simulink model "AXI_QPSK_Tx"  (R2023b)
settings: Solver=FixedStepAuto  StartTime=0.0  StopTime=10/Rb  RelTol=1e-3
PreLoadFcn:
  | Rb = 1000;   % 1kbit / s
  | Rsym = Rb/2;   % 2 bits per symbol
  | Rsymbol = Rb/2;
  | OSR = 32;
  | f_error = 120;
  | 
  | design_filters_tx
values from neighbouring files (symbols this model uses):
  CIC_fine_Tx = 2^-(CIC_right_shift - CIC_left_shift - CIC_shift_Tx)    [design_filters_tx.m]
  fCIC = fCICcomp * R_CIC    (= 25600000)    [design_filters_tx.m]
  fHB = fRRC * R_HB    (= 4000)    [design_filters_tx.m]
  R_CIC = 3200    [design_filters_tx.m]
  R_CICcomp = 2    [design_filters_tx.m]
  R_HB = 2    [design_filters_tx.m]
  R_RRC = 4    [design_filters_tx.m]
undefined symbols (not defined in the file or in its folder): AXI4, Lite
libraries: hdlBasic x309, hdlDSPIP x8, hdlsllib x2, vmcUtilities x1
(part 1 of 3)
CloseFcn:
  | clear
settings Model: Creator=nas07122  LastModifiedBy=Jakub
settings SolverCC: AlgebraicLoopSolver=TrustRegion
settings DataIOCC: ReturnWorkspaceOutputs=off
settings DebuggingCC: UnconnectedInputMsg=warning  UnconnectedOutputMsg=warning  UnconnectedLineMsg=warning  ArithmeticOperatorsInVariantConditions=warning
settings ModelReferenceCC: EnableRefExpFcnMdlSchedulingChecks=on
settings SFSimCC: SimUseLocalCustomCode=off  CustomCodeUndefinedFunction=UseInterfaceOnly
settings RTWCC: RTWUseLocalCustomCode=off
settings CodeAppCC: StateflowObjectComments=on

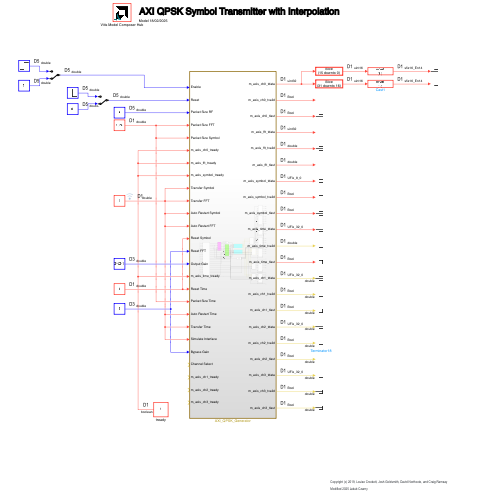
[thumbnail: Simulink's stored preview of the top-level diagram]
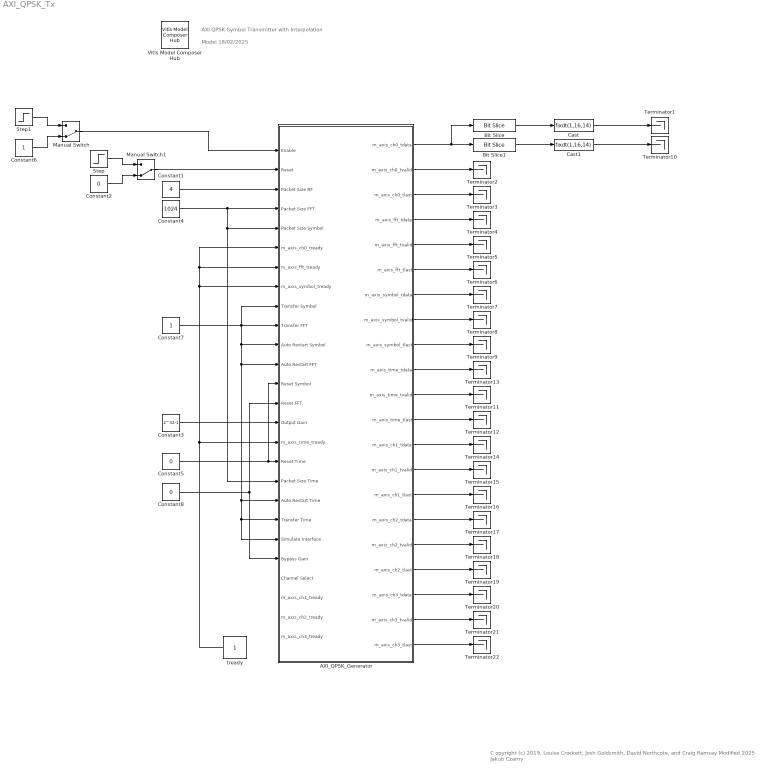
== system AXI_QPSK_Tx ==
  note: Model 18/02/2025
  note: AXI QPSK Symbol Transmitter with Interpolation
  note: C opyright (c) 2019, Louise Crockett, Josh Goldsmith, David Northcote, and Craig Ramsay
      | Modified 2025 Jakub Czarny
  AXI_QPSK_Generator : Subsystem
  Bit Slice : hdlsllib/Logic and Bit Operations/Bit Slice  lidx=15  ridx=0
  Bit Slice1 : hdlsllib/Logic and Bit Operations/Bit Slice  lidx=31  ridx=16
  Cast : DataTypeConversion  OutDataTypeStr=fixdt(1,16,14)  ConvertRealWorld=Stored Integer (SI)  SaturateOnIntegerOverflow=off  RndMeth=Floor
  Cast1 : DataTypeConversion  OutDataTypeStr=fixdt(1,16,14)  ConvertRealWorld=Stored Integer (SI)  SaturateOnIntegerOverflow=off  RndMeth=Floor
  Constant1 : Constant  Value=4  SampleTime=2/Rb
  Constant2 : Constant  Value=0  SampleTime=2/Rb
  Constant3 : Constant  Value=2^32-1  SampleTime=1/fHB
  Constant4 : Constant  Value=1024  SampleTime=1/fCIC
  Constant5 : Constant  Value=0  SampleTime=1/fCIC
  Constant6 : Constant  SampleTime=2/Rb
  Constant7 : Constant  SampleTime=1/fCIC
  Constant8 : Constant  Value=0  SampleTime=1/fHB
  Manual Switch : ManualSwitch  CurrentSetting=0
  Manual Switch1 : ManualSwitch  CurrentSetting=0
  Step : Step  Time=5/Rb  Before=1  After=0  SampleTime=2/Rb
  Step1 : Step  Time=8/Rb  SampleTime=2/Rb
  Terminator{1..22} (22 alike) : Terminator
  Vitis Model Composer Hub : vmcUtilities/Vitis Model Composer Hub  Tag=genX  CodeGeneration=off  SubsystemName=AXI_QPSK_Tx  CompilationType=HDLCompilation  ExportTypeV2=IP Catalog  TargetDirectory=../iprepo/zcu111/tx  exportDesign=off  analyzeDesign=off  validateDesignOnHw=off  ExportType=System Generator  IpVendor=xilinx.com  IpLibrary=hls  IpVersion=1.0  IpHWLanguage=Verilog  AieCompilerOptions={}  AieSimulatorOptions={}  CreateTestbench=off  TestbenchStackSize=10  RunRtlSim=off  RunCSim=off  RunAieSim=off  AieSimTimeout=50000  RunAieSimProfiling=off  LaunchVitisAnalyzer=off  PlotOutput=off  RunX86Sim=off  X86SimTimeout=10  GenHwImage=off  GenLibadfXo=on  GenHwValidationCode=off  PlatformType=Not Specified  HwSystemType=Baremetal  HwValidationTarget=hw  ProjDevice=xczu28dr-ffvg1517-2-e  ProjDevicePart=xczu28dr-ffvg1517-2-e  SamplePeriod=-1  ClockFrequency=200  DataPathParallelism=1  xilinxfamily=zynquplusRFSOC  part=xczu28dr  speed=-2-e  package=ffvg1517  directory=../iprepo/zcu111/tx\ip\AXI_QPSK_Tx\src  testbench=off  incr_netlist=off  synthesis_tool=Vivado  clock_wrapper=Clock Enables  dbl_ovrd=According to Block Masks  dcm_input_clock_period=10  sysclk_period=(1/fCIC)*1e9  simulink_period=1/(0.5*Rb*R_RRC*R_HB*R_CICcomp*R_CIC)  eval_field=0  LogFileName=''  NThreads=4
  tready : Constant  VectorParams1D=off  OutDataTypeStr=boolean  SampleTime=-1
  wires:
  Step1/1 -> Manual Switch/1
  Constant6/1 -> Manual Switch/2
  Bit Slice/1 -> Cast/1
  Bit Slice1/1 -> Cast1/1
  AXI_QPSK_Generator/1(m_axis_ch0_tdata) -> Bit Slice/1, Bit Slice1/1
  Manual Switch/1 -> AXI_QPSK_Generator/1(Enable)
  Constant1/1 -> AXI_QPSK_Generator/3(Packet Size RF)
  tready/1 -> AXI_QPSK_Generator/7(m_axis_fft_tready), AXI_QPSK_Generator/6(m_axis_ch0_tready), AXI_QPSK_Generator/8(m_axis_symbol_tready), AXI_QPSK_Generator/16(m_axis_time_tready)
  Manual Switch1/1 -> AXI_QPSK_Generator/2(Reset)
  Step/1 -> Manual Switch1/1
  Constant2/1 -> Manual Switch1/2
  Constant4/1 -> AXI_QPSK_Generator/5(Packet Size Symbol), AXI_QPSK_Generator/18(Packet Size Time), AXI_QPSK_Generator/4(Packet Size FFT)
  Constant5/1 -> AXI_QPSK_Generator/13(Reset Symbol), AXI_QPSK_Generator/17(Reset Time)
  Constant7/1 -> AXI_QPSK_Generator/21(Simulate Interface), AXI_QPSK_Generator/20(Transfer Time), AXI_QPSK_Generator/19(Auto Restart Time), AXI_QPSK_Generator/12(Auto Restart FFT), AXI_QPSK_Generator/11(Auto Restart Symbol), AXI_QPSK_Generator/10(Transfer FFT), AXI_QPSK_Generator/9(Transfer Symbol)
  Constant8/1 -> AXI_QPSK_Generator/14(Reset FFT), AXI_QPSK_Generator/22(Bypass Gain)
  Constant3/1 -> AXI_QPSK_Generator/15(Output Gain)
  AXI_QPSK_Generator/2(m_axis_ch0_tvalid) -> Terminator2/1
  AXI_QPSK_Generator/3(m_axis_ch0_tlast) -> Terminator3/1
  AXI_QPSK_Generator/5(m_axis_fft_tvalid) -> Terminator5/1
  AXI_QPSK_Generator/4(m_axis_fft_tdata) -> Terminator4/1
  AXI_QPSK_Generator/8(m_axis_symbol_tvalid) -> Terminator8/1
  AXI_QPSK_Generator/9(m_axis_symbol_tlast) -> Terminator9/1
  AXI_QPSK_Generator/7(m_axis_symbol_tdata) -> Terminator7/1
  AXI_QPSK_Generator/6(m_axis_fft_tlast) -> Terminator6/1
  AXI_QPSK_Generator/12(m_axis_time_tlast) -> Terminator12/1
  AXI_QPSK_Generator/10(m_axis_time_tdata) -> Terminator13/1
  Cast/1 -> Terminator1/1
  Cast1/1 -> Terminator10/1
  AXI_QPSK_Generator/11(m_axis_time_tvalid) -> Terminator11/1
  AXI_QPSK_Generator/13(m_axis_ch1_tdata) -> Terminator14/1
  AXI_QPSK_Generator/14(m_axis_ch1_tvalid) -> Terminator15/1
  AXI_QPSK_Generator/15(m_axis_ch1_tlast) -> Terminator16/1
  AXI_QPSK_Generator/16(m_axis_ch2_tdata) -> Terminator17/1
  AXI_QPSK_Generator/17(m_axis_ch2_tvalid) -> Terminator18/1
  AXI_QPSK_Generator/18(m_axis_ch2_tlast) -> Terminator19/1
  AXI_QPSK_Generator/19(m_axis_ch3_tdata) -> Terminator20/1
  AXI_QPSK_Generator/20(m_axis_ch3_tvalid) -> Terminator21/1
  AXI_QPSK_Generator/21(m_axis_ch3_tlast) -> Terminator22/1

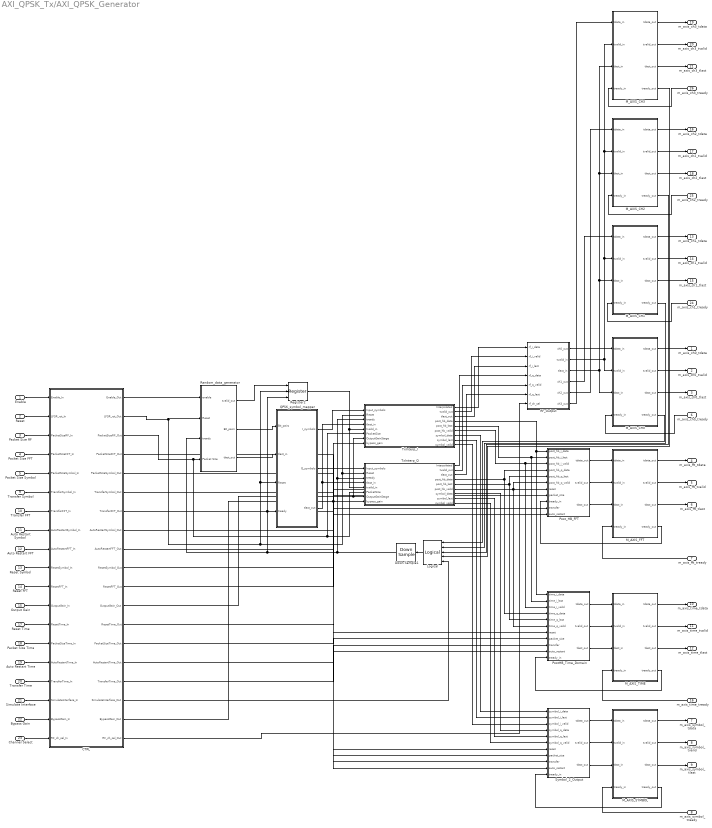
== system AXI_QPSK_Tx/AXI_QPSK_Generator ==
  Enable : Inport
  Reset : Inport  Port=2
  Packet Size RF : Inport  Port=3
  Packet Size FFT : Inport  Port=4
  Packet Size Symbol : Inport  Port=5
  m_axis_ch0_tready : Inport  Port=6
  m_axis_fft_tready : Inport  Port=7
  m_axis_symbol_tready : Inport  Port=8
  Transfer Symbol : Inport  Port=9
  Transfer FFT : Inport  Port=10
  Auto Restart Symbol : Inport  Port=11
  Auto Restart FFT : Inport  Port=12
  Reset Symbol : Inport  Port=13
  Reset FFT : Inport  Port=14
  Output Gain : Inport  Port=15
  m_axis_time_tready : Inport  Port=16
  Reset Time : Inport  Port=17
  Packet Size Time : Inport  Port=18
  Auto Restart Time : Inport  Port=19
  Transfer Time : Inport  Port=20
  Simulate Interface : Inport  Port=21
  Bypass Gain : Inport  Port=22
  Channel Select : Inport  Port=23
  m_axis_ch1_tready : Inport  Port=24
  m_axis_ch2_tready : Inport  Port=25
  m_axis_ch3_tready : Inport  Port=26
  CTRL : Subsystem
  Down Sample1 : hdlBasic/Down Sample  sample_ratio=fCIC/(Rb/2)  sample_phase=First Value of Frame  en=off  rst=off  latency=0  XmcBlockStatus=1  maskContainerNames=group1  block_type=dsamp  block_config=sysgen:Downsample_config
  Logical : hdlBasic/Logical  logical_function=OR  inputs=5  en=off  latency=0  precision=Full  arith_type=Unsigned  n_bits=16  bin_pt=0  align_bp=on  overflow=[]  quantization=[]  XmcBlockStatus=1  maskContainerNames=tabcontainer1  block_type=logical  block_config=sysgen:Logical_config
  M_AXIS_CH0 : Subsystem
  M_AXIS_CH1 : Subsystem
  M_AXIS_CH2 : Subsystem
  M_AXIS_CH3 : Subsystem
  M_AXIS_FFT : Subsystem
  M_AXIS_SYMBOL : Subsystem
  M_AXIS_TIME : Subsystem
  PostHB_Time_Domain : Subsystem
  Post_HB_FFT : Subsystem
  QPSK_symbol_mapper : Subsystem
  RF_Output : Subsystem
  Random_data_generator : Subsystem
  Register2 : hdlBasic/Register  init=0  rst=on  en=on  XmcBlockStatus=1  maskContainerNames=tabcontainer1  block_type=register  block_config=sysgen:Register_config
  Symbol_2_Output : Subsystem
  TxInterp_I : Subsystem
  TxInterp_Q : Subsystem
  m_axis_ch0_tdata : Outport  VectorParamsAs1DForOutWhenUnconnected=off
  m_axis_ch0_tvalid : Outport  Port=2  VectorParamsAs1DForOutWhenUnconnected=off
  m_axis_ch0_tlast : Outport  Port=3  VectorParamsAs1DForOutWhenUnconnected=off
  m_axis_fft_tdata : Outport  Port=4  VectorParamsAs1DForOutWhenUnconnected=off
  m_axis_fft_tvalid : Outport  Port=5  VectorParamsAs1DForOutWhenUnconnected=off
  m_axis_fft_tlast : Outport  Port=6  VectorParamsAs1DForOutWhenUnconnected=off
  m_axis_symbol_tdata : Outport  Port=7  VectorParamsAs1DForOutWhenUnconnected=off
  m_axis_symbol_tvalid : Outport  Port=8  VectorParamsAs1DForOutWhenUnconnected=off
  m_axis_symbol_tlast : Outport  Port=9  VectorParamsAs1DForOutWhenUnconnected=off
  m_axis_time_tdata : Outport  Port=10  VectorParamsAs1DForOutWhenUnconnected=off
  m_axis_time_tvalid : Outport  Port=11  VectorParamsAs1DForOutWhenUnconnected=off
  m_axis_time_tlast : Outport  Port=12  VectorParamsAs1DForOutWhenUnconnected=off
  m_axis_ch1_tdata : Outport  Port=13  VectorParamsAs1DForOutWhenUnconnected=off
  m_axis_ch1_tvalid : Outport  Port=14  VectorParamsAs1DForOutWhenUnconnected=off
  m_axis_ch1_tlast : Outport  Port=15  VectorParamsAs1DForOutWhenUnconnected=off
  m_axis_ch2_tdata : Outport  Port=16  VectorParamsAs1DForOutWhenUnconnected=off
  m_axis_ch2_tvalid : Outport  Port=17  VectorParamsAs1DForOutWhenUnconnected=off
  m_axis_ch2_tlast : Outport  Port=18  VectorParamsAs1DForOutWhenUnconnected=off
  m_axis_ch3_tdata : Outport  Port=19  VectorParamsAs1DForOutWhenUnconnected=off
  m_axis_ch3_tvalid : Outport  Port=20  VectorParamsAs1DForOutWhenUnconnected=off
  m_axis_ch3_tlast : Outport  Port=21  VectorParamsAs1DForOutWhenUnconnected=off
  wires:
  QPSK_symbol_mapper/3(tlast_out) -> TxInterp_I/4(tlast_in), TxInterp_Q/4(tlast_in)
  M_AXIS_CH0/2(tvalid_out) -> m_axis_ch0_tvalid/1
  QPSK_symbol_mapper/1(I_symbols) -> TxInterp_I/1(Input_symbols)
  m_axis_ch0_tready/1 -> M_AXIS_CH0/4(tready_in)
  QPSK_symbol_mapper/2(Q_symbols) -> TxInterp_Q/1(Input_symbols)
  Packet Size RF/1 -> CTRL/3(PacketSizeRF_In)
  Reset/1 -> CTRL/2(LFSR_rst_In)
  Random_data_generator/3(tlast_out) -> QPSK_symbol_mapper/2(tlast_in)
  Enable/1 -> CTRL/1(Enable_In)
  Random_data_generator/2(Bit_pairs) -> QPSK_symbol_mapper/1(Bit_pairs)
  CTRL/3(PacketSizeRF_Out) -> TxInterp_I/6(PacketSize), TxInterp_Q/6(PacketSize), Random_data_generator/4(Packet Size)
  M_AXIS_CH0/3(tlast_out) -> m_axis_ch0_tlast/1
  M_AXIS_CH0/1(tdata_out) -> m_axis_ch0_tdata/1
  Down Sample1/1 -> Random_data_generator/3(tready), Register2/3, QPSK_symbol_mapper/4(tready), TxInterp_I/3(tready), TxInterp_Q/3(tready)
  CTRL/2(LFSR_rst_Out) -> Random_data_generator/2(Reset), TxInterp_I/2(Reset), TxInterp_Q/2(Reset), QPSK_symbol_mapper/3(Reset), Register2/2
  CTRL/1(Enable_Out) -> Random_data_generator/1(enable)
  Random_data_generator/1(tvalid_out) -> Register2/1
  Register2/1 -> TxInterp_I/5(tvalid_in), TxInterp_Q/5(tvalid_in)
  Post_HB_FFT/1(tdata_out) -> M_AXIS_FFT/1(tdata_in)
  Post_HB_FFT/2(tvalid_out) -> M_AXIS_FFT/2(tvalid_in)
  Post_HB_FFT/3(tlast_out) -> M_AXIS_FFT/3(tlast_in)
  M_AXIS_FFT/1(tdata_out) -> m_axis_fft_tdata/1
  M_AXIS_FFT/3(tlast_out) -> m_axis_fft_tlast/1
  m_axis_fft_tready/1 -> M_AXIS_FFT/4(tready_in)
  M_AXIS_FFT/2(tvalid_out) -> m_axis_fft_tvalid/1
  M_AXIS_SYMBOL/2(tvalid_out) -> m_axis_symbol_tvalid/1
  m_axis_symbol_tready/1 -> M_AXIS_SYMBOL/4(tready_in)
  M_AXIS_SYMBOL/3(tlast_out) -> m_axis_symbol_tlast/1
  M_AXIS_SYMBOL/1(tdata_out) -> m_axis_symbol_tdata/1
  TxInterp_I/4(post_hb_data) -> PostHB_Time_Domain/1(time_i_data), Post_HB_FFT/1(post_hb_i_data)
  TxInterp_I/5(post_hb_last) -> PostHB_Time_Domain/2(time_i_last), Post_HB_FFT/2(post_hb_i_last)
  TxInterp_I/6(post_hb_valid) -> PostHB_Time_Domain/3(time_i_valid), Post_HB_FFT/3(post_hb_i_valid)
  Symbol_2_Output/1(tdata_out) -> M_AXIS_SYMBOL/1(tdata_in)
  Symbol_2_Output/2(tvalid_out) -> M_AXIS_SYMBOL/2(tvalid_in)
  Symbol_2_Output/3(tlast_out) -> M_AXIS_SYMBOL/3(tlast_in)
  M_AXIS_SYMBOL/4(tready_out) -> Symbol_2_Output/11(tready_in)
  M_AXIS_FFT/4(tready_out) -> Post_HB_FFT/9(tready_in)
  TxInterp_I/1(Interpolated) -> RF_Output/1(rf_i_data)
  TxInterp_I/2(tvalid_out) -> RF_Output/2(rf_i_valid)
  TxInterp_I/3(tlast_out) -> RF_Output/3(rf_i_last)
  RF_Output/1(ch0_out) -> M_AXIS_CH0/1(tdata_in)
  RF_Output/2(tvalid_in) -> M_AXIS_CH0/2(tvalid_in), M_AXIS_CH3/2(tvalid_in), M_AXIS_CH2/2(tvalid_in), M_AXIS_CH1/2(tvalid_in)
  RF_Output/3(tlast_in) -> M_AXIS_CH3/3(tlast_in), M_AXIS_CH2/3(tlast_in), M_AXIS_CH1/3(tlast_in), M_AXIS_CH0/3(tlast_in)
  TxInterp_I/7(symbol_data) -> Symbol_2_Output/1(symbol_i_data)
  TxInterp_I/8(symbol_last) -> Symbol_2_Output/2(symbol_i_last)
  TxInterp_I/9(symbol_valid) -> Symbol_2_Output/3(symbol_i_valid)
  CTRL/4(PacketSizeFFT_Out) -> Post_HB_FFT/8(packet_size)
  CTRL/5(PacketSizeSymbol_Out) -> Symbol_2_Output/8(packet_size)
  Packet Size FFT/1 -> CTRL/4(PacketSizeFFT_In)
  Packet Size Symbol/1 -> CTRL/5(PacketSizeSymbol_In)
  CTRL/6(TransferSymbol_Out) -> Symbol_2_Output/9(transfer)
  CTRL/8(AutoRestartSymbol_Out) -> Symbol_2_Output/10(auto_restart)
  CTRL/10(ResetSymbol_Out) -> Symbol_2_Output/7(reset)
  Transfer Symbol/1 -> CTRL/6(TransferSymbol_In)
  Transfer FFT/1 -> CTRL/7(TransferFFT_In)
  Auto Restart Symbol/1 -> CTRL/8(AutoRestartSymbol_In)
  Auto Restart FFT/1 -> CTRL/9(AutoRestartFFT_In)
  Reset Symbol/1 -> CTRL/10(ResetSymbol_In)
  Reset FFT/1 -> CTRL/11(ResetFFT_In)
  CTRL/7(TransferFFT_Out) -> Post_HB_FFT/10(transfer)
  CTRL/9(AutoRestartFFT_Out) -> Post_HB_FFT/11(auto_restart)
  CTRL/11(ResetFFT_Out) -> Post_HB_FFT/7(reset)
  CTRL/12(OutputGain_Out) -> TxInterp_I/7(OutputGainStage), TxInterp_Q/7(OutputGainStage)
  Output Gain/1 -> CTRL/12(OutputGain_In)
  M_AXIS_TIME/4(tready_out) -> PostHB_Time_Domain/11(tready_in)
  PostHB_Time_Domain/3(tlast_out) -> M_AXIS_TIME/3(tlast_in)
  PostHB_Time_Domain/2(tvalid_out) -> M_AXIS_TIME/2(tvalid_in)
  PostHB_Time_Domain/1(tdata_out) -> M_AXIS_TIME/1(tdata_in)
  M_AXIS_TIME/1(tdata_out) -> m_axis_time_tdata/1
  M_AXIS_TIME/3(tlast_out) -> m_axis_time_tlast/1
  m_axis_time_tready/1 -> M_AXIS_TIME/4(tready_in)
  M_AXIS_TIME/2(tvalid_out) -> m_axis_time_tvalid/1
  CTRL/13(ResetTime_Out) -> PostHB_Time_Domain/7(reset)
  CTRL/14(PacketSizeTime_Out) -> PostHB_Time_Domain/8(packet_size)
  CTRL/15(AutoRestartTime_Out) -> PostHB_Time_Domain/10(auto_restart)
  CTRL/16(TransferTime_Out) -> PostHB_Time_Domain/9(transfer)
  Reset Time/1 -> CTRL/13(ResetTime_In)
  Packet Size Time/1 -> CTRL/14(PacketSizeTime_In)
  Auto Restart Time/1 -> CTRL/15(AutoRestartTime_In)
  Transfer Time/1 -> CTRL/16(TransferTime_In)
  M_AXIS_CH0/4(tready_out) -> Logical/1
  Logical/1 -> Down Sample1/1
  CTRL/17(SimulateInterface_Out) -> Logical/5
  Simulate Interface/1 -> CTRL/17(SimulateInterface_In)
  CTRL/18(BypassGain_Out) -> TxInterp_I/8(bypass_gain), TxInterp_Q/8(bypass_gain)
  TxInterp_Q/1(Interpolated) -> RF_Output/4(rf_q_data)
  TxInterp_Q/2(tvalid_out) -> RF_Output/5(rf_q_valid)
  TxInterp_Q/3(tlast_out) -> RF_Output/6(rf_q_last)
  TxInterp_Q/4(post_hb_data) -> PostHB_Time_Domain/4(time_q_data), Post_HB_FFT/4(post_hb_q_data)
  TxInterp_Q/5(post_hb_last) -> PostHB_Time_Domain/5(time_q_last), Post_HB_FFT/5(post_hb_q_last)
  TxInterp_Q/6(post_hb_valid) -> PostHB_Time_Domain/6(time_q_valid), Post_HB_FFT/6(post_hb_q_valid)
  TxInterp_Q/7(symbol_data) -> Symbol_2_Output/4(symbol_q_data)
  TxInterp_Q/8(symbol_last) -> Symbol_2_Output/5(symbol_q_last)
  TxInterp_Q/9(symbol_valid) -> Symbol_2_Output/6(symbol_q_valid)
  Bypass Gain/1 -> CTRL/18(BypassGain_In)
  Channel Select/1 -> CTRL/19(RF_ch_sel_In)
  CTRL/19(RF_ch_sel_Out) -> RF_Output/7(rf_ch_sel)
  M_AXIS_CH1/3(tlast_out) -> m_axis_ch1_tlast/1
  M_AXIS_CH1/1(tdata_out) -> m_axis_ch1_tdata/1
  m_axis_ch1_tready/1 -> M_AXIS_CH1/4(tready_in)
  M_AXIS_CH1/2(tvalid_out) -> m_axis_ch1_tvalid/1
  M_AXIS_CH1/4(tready_out) -> Logical/2
  RF_Output/4(ch1_out) -> M_AXIS_CH1/1(tdata_in)
  M_AXIS_CH2/2(tvalid_out) -> m_axis_ch2_tvalid/1
  M_AXIS_CH2/1(tdata_out) -> m_axis_ch2_tdata/1
  m_axis_ch2_tready/1 -> M_AXIS_CH2/4(tready_in)
  M_AXIS_CH2/3(tlast_out) -> m_axis_ch2_tlast/1
  RF_Output/5(ch2_out) -> M_AXIS_CH2/1(tdata_in)
  M_AXIS_CH2/4(tready_out) -> Logical/3
  m_axis_ch3_tready/1 -> M_AXIS_CH3/4(tready_in)
  M_AXIS_CH3/1(tdata_out) -> m_axis_ch3_tdata/1
  M_AXIS_CH3/2(tvalid_out) -> m_axis_ch3_tvalid/1
  M_AXIS_CH3/3(tlast_out) -> m_axis_ch3_tlast/1
  M_AXIS_CH3/4(tready_out) -> Logical/4
  RF_Output/6(ch3_out) -> M_AXIS_CH3/1(tdata_in)

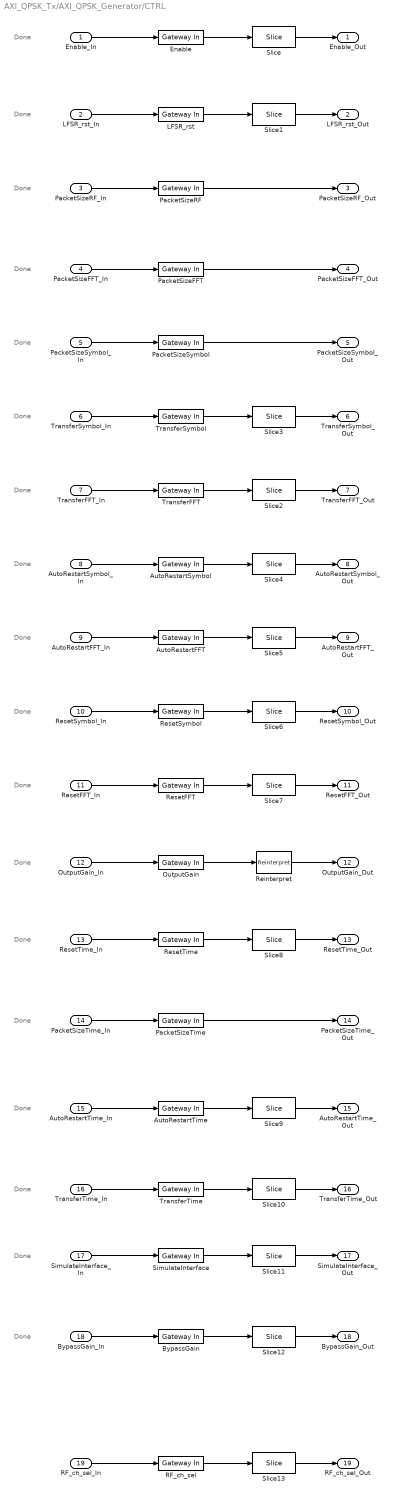
== system AXI_QPSK_Tx/AXI_QPSK_Generator/CTRL ==
  note: Done
  note: Done
  note: Done
  note: Done
  note: Done
  note: Done
  note: Done
  note: Done
  note: Done
  note: Done
  note: Done
  note: Done
  note: Done
  note: Done
  note: Done
  note: Done
  note: Done
  note: Done
  Enable_In : Inport
  LFSR_rst_In : Inport  Port=2
  PacketSizeRF_In : Inport  Port=3
  PacketSizeFFT_In : Inport  Port=4
  PacketSizeSymbol_In : Inport  Port=5
  TransferSymbol_In : Inport  Port=6
  TransferFFT_In : Inport  Port=7
  AutoRestartSymbol_In : Inport  Port=8
  AutoRestartFFT_In : Inport  Port=9
  ResetSymbol_In : Inport  Port=10
  ResetFFT_In : Inport  Port=11
  OutputGain_In : Inport  Port=12
  ResetTime_In : Inport  Port=13
  PacketSizeTime_In : Inport  Port=14
  AutoRestartTime_In : Inport  Port=15
  TransferTime_In : Inport  Port=16
  SimulateInterface_In : Inport  Port=17
  BypassGain_In : Inport  Port=18
  RF_ch_sel_In : Inport  Port=19
  AutoRestartFFT : hdlBasic/Gateway In  gui_display_data_type=Fixed-point  arith_type=Unsigned  n_bits=32  bin_pt=0  preci_type=Single  exp_width=8  frac_width=24  rows=1  columns=1  quantization=Truncate  overflow=Wrap  period=1/fCIC  UseAsADC=off  ADCChannel='1'  interface=AXI4-Lite  automatic_assignment=off  address_offset=40  intf_name=''  intf_description=''  default_value=0  timing_constraint=None  locs_specified=off  LOCs={}  io_standard={}  inherit_from_input=off  hdl_port=on  XmcBlockStatus=1  maskContainerNames=group4  block_type=gatewayin  block_config=sysgen:gateway_in_config  block_width_w=590  block_height_w=620  block_width=640  block_height=850
  AutoRestartSymbol : hdlBasic/Gateway In  gui_display_data_type=Fixed-point  arith_type=Unsigned  n_bits=32  bin_pt=0  preci_type=Single  exp_width=8  frac_width=24  rows=1  columns=1  quantization=Truncate  overflow=Wrap  period=1/fCIC  UseAsADC=off  ADCChannel='1'  interface=AXI4-Lite  automatic_assignment=off  address_offset=36  intf_name=''  intf_description=''  default_value=0  timing_constraint=None  locs_specified=off  LOCs={}  io_standard={}  inherit_from_input=off  hdl_port=on  XmcBlockStatus=1  maskContainerNames=group4  block_type=gatewayin  block_config=sysgen:gateway_in_config  block_width_w=590  block_height_w=620  block_width=640  block_height=850
  AutoRestartTime : hdlBasic/Gateway In  gui_display_data_type=Fixed-point  arith_type=Unsigned  n_bits=32  bin_pt=0  preci_type=Single  exp_width=8  frac_width=24  rows=1  columns=1  quantization=Truncate  overflow=Wrap  period=1/fCIC  UseAsADC=off  ADCChannel='1'  interface=AXI4-Lite  automatic_assignment=off  address_offset=56  intf_name=''  intf_description=''  default_value=0  timing_constraint=None  locs_specified=off  LOCs={}  io_standard={}  inherit_from_input=off  hdl_port=on  XmcBlockStatus=1  maskContainerNames=group4  block_type=gatewayin  block_config=sysgen:gateway_in_config  block_width_w=590  block_height_w=620  block_width=640  block_height=850
  BypassGain : hdlBasic/Gateway In  gui_display_data_type=Fixed-point  arith_type=Unsigned  n_bits=32  bin_pt=0  preci_type=Single  exp_width=8  frac_width=24  rows=1  columns=1  quantization=Truncate  overflow=Wrap  period=1/fHB  UseAsADC=off  ADCChannel='1'  interface=AXI4-Lite  automatic_assignment=off  address_offset=68  intf_name=''  intf_description=''  default_value=0  timing_constraint=None  locs_specified=off  LOCs={}  io_standard={}  inherit_from_input=off  hdl_port=on  XmcBlockStatus=1  maskContainerNames=group4  block_type=gatewayin  block_config=sysgen:gateway_in_config  block_width_w=590  block_height_w=620  block_width=640  block_height=850
  Enable : hdlBasic/Gateway In  gui_display_data_type=Fixed-point  arith_type=Unsigned  n_bits=32  bin_pt=0  preci_type=Single  exp_width=8  frac_width=24  rows=1  columns=1  quantization="Round  (unbiased: +/- Inf)"  overflow=Saturate  period=2/Rb  UseAsADC=off  ADCChannel='1'  interface=AXI4-Lite  automatic_assignment=off  address_offset=32  intf_name=''  intf_description=''  default_value=0  timing_constraint=None  locs_specified=off  LOCs={}  io_standard={}  inherit_from_input=off  hdl_port=on  XmcBlockStatus=1  maskContainerNames=group4  block_type=gatewayin  block_config=sysgen:gateway_in_config  block_width_w=590  block_height_w=620  block_width=640  block_height=850
  LFSR_rst : hdlBasic/Gateway In  gui_display_data_type=Fixed-point  arith_type=Unsigned  n_bits=32  bin_pt=0  preci_type=Single  exp_width=8  frac_width=24  rows=1  columns=1  quantization="Round  (unbiased: +/- Inf)"  overflow=Saturate  period=2/Rb  UseAsADC=off  ADCChannel='1'  interface=AXI4-Lite  automatic_assignment=off  address_offset=28  intf_name=''  intf_description=''  default_value=0  timing_constraint=None  locs_specified=off  LOCs={}  io_standard={}  inherit_from_input=off  hdl_port=on  XmcBlockStatus=1  maskContainerNames=group4  block_type=gatewayin  block_config=sysgen:gateway_in_config  block_width_w=590  block_height_w=620  block_width=640  block_height=850
  OutputGain : hdlBasic/Gateway In  gui_display_data_type=Fixed-point  arith_type=Unsigned  n_bits=32  bin_pt=0  preci_type=Single  exp_width=8  frac_width=24  rows=1  columns=1  quantization=Truncate  overflow=Wrap  period=1/fHB  UseAsADC=off  ADCChannel='1'  interface=AXI4-Lite  automatic_assignment=off  address_offset=44  intf_name=''  intf_description=''  default_value=0  timing_constraint=None  locs_specified=off  LOCs={}  io_standard={}  inherit_from_input=off  hdl_port=on  XmcBlockStatus=1  maskContainerNames=group4  block_type=gatewayin  block_config=sysgen:gateway_in_config  block_width_w=590  block_height_w=620  block_width=640  block_height=850
  PacketSizeFFT : hdlBasic/Gateway In  gui_display_data_type=Fixed-point  arith_type=Unsigned  n_bits=32  bin_pt=0  preci_type=Single  exp_width=8  frac_width=24  rows=1  columns=1  quantization=Truncate  overflow=Wrap  period=1/fCIC  UseAsADC=off  ADCChannel='1'  interface=AXI4-Lite  automatic_assignment=off  address_offset=24  intf_name=''  intf_description=''  default_value=0  timing_constraint=None  locs_specified=off  LOCs={}  io_standard={}  inherit_from_input=off  hdl_port=on  XmcBlockStatus=1  maskContainerNames=group4  block_type=gatewayin  block_config=sysgen:gateway_in_config  block_width_w=590  block_height_w=620  block_width=640  block_height=850
  PacketSizeRF : hdlBasic/Gateway In  gui_display_data_type=Fixed-point  arith_type=Unsigned  n_bits=32  bin_pt=0  preci_type=Single  exp_width=8  frac_width=24  rows=1  columns=1  quantization=Truncate  overflow=Wrap  period=2/Rb  UseAsADC=off  ADCChannel='1'  interface=AXI4-Lite  automatic_assignment=off  address_offset=20  intf_name=''  intf_description=''  default_value=0  timing_constraint=None  locs_specified=off  LOCs={}  io_standard={}  inherit_from_input=off  hdl_port=on  XmcBlockStatus=1  maskContainerNames=group4  block_type=gatewayin  block_config=sysgen:gateway_in_config  block_width_w=590  block_height_w=620  block_width=640  block_height=850
  PacketSizeSymbol : hdlBasic/Gateway In  gui_display_data_type=Fixed-point  arith_type=Unsigned  n_bits=32  bin_pt=0  preci_type=Single  exp_width=8  frac_width=24  rows=1  columns=1  quantization=Truncate  overflow=Wrap  period=1/fCIC  UseAsADC=off  ADCChannel='1'  interface=AXI4-Lite  automatic_assignment=off  address_offset=16  intf_name=''  intf_description=''  default_value=0  timing_constraint=None  locs_specified=off  LOCs={}  io_standard={}  inherit_from_input=off  hdl_port=on  XmcBlockStatus=1  maskContainerNames=group4  block_type=gatewayin  block_config=sysgen:gateway_in_config  block_width_w=590  block_height_w=620  block_width=640  block_height=850
  PacketSizeTime : hdlBasic/Gateway In  gui_display_data_type=Fixed-point  arith_type=Unsigned  n_bits=32  bin_pt=0  preci_type=Single  exp_width=8  frac_width=24  rows=1  columns=1  quantization=Truncate  overflow=Wrap  period=1/fCIC  UseAsADC=off  ADCChannel='1'  interface=AXI4-Lite  automatic_assignment=off  address_offset=52  intf_name=''  intf_description=''  default_value=0  timing_constraint=None  locs_specified=off  LOCs={}  io_standard={}  inherit_from_input=off  hdl_port=on  XmcBlockStatus=1  maskContainerNames=group4  block_type=gatewayin  block_config=sysgen:gateway_in_config  block_width_w=590  block_height_w=620  block_width=640  block_height=850
  RF_ch_sel : hdlBasic/Gateway In  gui_display_data_type=Fixed-point  arith_type=Unsigned  n_bits=32  bin_pt=0  preci_type=Single  exp_width=8  frac_width=24  rows=1  columns=1  quantization="Round  (unbiased: +/- Inf)"  overflow=Saturate  period=2/Rb  UseAsADC=off  ADCChannel='1'  interface=AXI4-Lite  automatic_assignment=off  address_offset=72  intf_name=''  intf_description=''  default_value=0  timing_constraint=None  locs_specified=off  LOCs={}  io_standard={}  inherit_from_input=off  hdl_port=on  XmcBlockStatus=1  maskContainerNames=group4  block_type=gatewayin  block_config=sysgen:gateway_in_config  block_width_w=590  block_height_w=620  block_width=640  block_height=850
  Reinterpret : hdlBasic/Reinterpret  force_arith_type=off  arith_type=Unsigned  force_bin_pt=on  bin_pt=32  XmcBlockStatus=1  maskContainerNames=group1  block_type=reinterpret  block_config=sysgen:Reinterpret_config
  ResetFFT : hdlBasic/Gateway In  gui_display_data_type=Fixed-point  arith_type=Unsigned  n_bits=32  bin_pt=0  preci_type=Single  exp_width=8  frac_width=24  rows=1  columns=1  quantization=Truncate  overflow=Wrap  period=1/fHB  UseAsADC=off  ADCChannel='1'  interface=AXI4-Lite  automatic_assignment=off  address_offset=12  intf_name=''  intf_description=''  default_value=0  timing_constraint=None  locs_specified=off  LOCs={}  io_standard={}  inherit_from_input=off  hdl_port=on  XmcBlockStatus=1  maskContainerNames=group4  block_type=gatewayin  block_config=sysgen:gateway_in_config  block_width_w=590  block_height_w=620  block_width=640  block_height=850
  ResetSymbol : hdlBasic/Gateway In  gui_display_data_type=Fixed-point  arith_type=Unsigned  n_bits=32  bin_pt=0  preci_type=Single  exp_width=8  frac_width=24  rows=1  columns=1  quantization=Truncate  overflow=Wrap  period=1/fCIC  UseAsADC=off  ADCChannel='1'  interface=AXI4-Lite  automatic_assignment=off  address_offset=8  intf_name=''  intf_description=''  default_value=0  timing_constraint=None  locs_specified=off  LOCs={}  io_standard={}  inherit_from_input=off  hdl_port=on  XmcBlockStatus=1  maskContainerNames=group4  block_type=gatewayin  block_config=sysgen:gateway_in_config  block_width_w=590  block_height_w=620  block_width=640  block_height=850
  ResetTime : hdlBasic/Gateway In  gui_display_data_type=Fixed-point  arith_type=Unsigned  n_bits=32  bin_pt=0  preci_type=Single  exp_width=8  frac_width=24  rows=1  columns=1  quantization=Truncate  overflow=Wrap  period=1/fCIC  UseAsADC=off  ADCChannel='1'  interface=AXI4-Lite  automatic_assignment=off  address_offset=48  intf_name=''  intf_description=''  default_value=0  timing_constraint=None  locs_specified=off  LOCs={}  io_standard={}  inherit_from_input=off  hdl_port=on  XmcBlockStatus=1  maskContainerNames=group4  block_type=gatewayin  block_config=sysgen:gateway_in_config  block_width_w=590  block_height_w=620  block_width=640  block_height=850
  SimulateInterface : hdlBasic/Gateway In  gui_display_data_type=Fixed-point  arith_type=Unsigned  n_bits=32  bin_pt=0  preci_type=Single  exp_width=8  frac_width=24  rows=1  columns=1  quantization=Truncate  overflow=Wrap  period=1/fCIC  UseAsADC=off  ADCChannel='1'  interface=AXI4-Lite  automatic_assignment=off  address_offset=64  intf_name=''  intf_description=''  default_value=0  timing_constraint=None  locs_specified=off  LOCs={}  io_standard={}  inherit_from_input=off  hdl_port=on  XmcBlockStatus=1  maskContainerNames=group4  block_type=gatewayin  block_config=sysgen:gateway_in_config  block_width_w=590  block_height_w=620  block_width=640  block_height=850
  Slice{,1..12} (13 alike) : hdlBasic/Slice  nbits=1  boolean_output=on  mode=Two Bit Locations  bit1=0  base1=LSB of Input  bit0=0  base0=LSB of Input  XmcBlockStatus=1  maskContainerNames=group1  block_type=slice  block_config=sysgen:Slice_config
  Slice13 : hdlBasic/Slice  nbits=2  boolean_output=off  mode=Lower Bit Location + Width  bit1=0  base1=LSB of Input  bit0=0  base0=LSB of Input  XmcBlockStatus=1  maskContainerNames=group1  block_type=slice  block_config=sysgen:Slice_config
  TransferFFT : hdlBasic/Gateway In  gui_display_data_type=Fixed-point  arith_type=Unsigned  n_bits=32  bin_pt=0  preci_type=Single  exp_width=8  frac_width=24  rows=1  columns=1  quantization=Truncate  overflow=Wrap  period=1/fCIC  UseAsADC=off  ADCChannel='1'  interface=AXI4-Lite  automatic_assignment=off  address_offset=4  intf_name=''  intf_description=''  default_value=0  timing_constraint=None  locs_specified=off  LOCs={}  io_standard={}  inherit_from_input=off  hdl_port=on  XmcBlockStatus=1  maskContainerNames=group4  block_type=gatewayin  block_config=sysgen:gateway_in_config  block_width_w=590  block_height_w=620  block_width=640  block_height=850
  TransferSymbol : hdlBasic/Gateway In  gui_display_data_type=Fixed-point  arith_type=Unsigned  n_bits=32  bin_pt=0  preci_type=Single  exp_width=8  frac_width=24  rows=1  columns=1  quantization=Truncate  overflow=Wrap  period=1/fCIC  UseAsADC=off  ADCChannel='1'  interface=AXI4-Lite  automatic_assignment=off  address_offset=0  intf_name=''  intf_description=''  default_value=0  timing_constraint=None  locs_specified=off  LOCs={}  io_standard={}  inherit_from_input=off  hdl_port=on  XmcBlockStatus=1  maskContainerNames=group4  block_type=gatewayin  block_config=sysgen:gateway_in_config  block_width_w=590  block_height_w=620  block_width=640  block_height=850
  TransferTime : hdlBasic/Gateway In  gui_display_data_type=Fixed-point  arith_type=Unsigned  n_bits=32  bin_pt=0  preci_type=Single  exp_width=8  frac_width=24  rows=1  columns=1  quantization=Truncate  overflow=Wrap  period=1/fCIC  UseAsADC=off  ADCChannel='1'  interface=AXI4-Lite  automatic_assignment=off  address_offset=60  intf_name=''  intf_description=''  default_value=0  timing_constraint=None  locs_specified=off  LOCs={}  io_standard={}  inherit_from_input=off  hdl_port=on  XmcBlockStatus=1  maskContainerNames=group4  block_type=gatewayin  block_config=sysgen:gateway_in_config  block_width_w=590  block_height_w=620  block_width=640  block_height=850
  Enable_Out : Outport  VectorParamsAs1DForOutWhenUnconnected=off
  LFSR_rst_Out : Outport  Port=2  VectorParamsAs1DForOutWhenUnconnected=off
  PacketSizeRF_Out : Outport  Port=3  VectorParamsAs1DForOutWhenUnconnected=off
  PacketSizeFFT_Out : Outport  Port=4  VectorParamsAs1DForOutWhenUnconnected=off
  PacketSizeSymbol_Out : Outport  Port=5  VectorParamsAs1DForOutWhenUnconnected=off
  TransferSymbol_Out : Outport  Port=6  VectorParamsAs1DForOutWhenUnconnected=off
  TransferFFT_Out : Outport  Port=7  VectorParamsAs1DForOutWhenUnconnected=off
  AutoRestartSymbol_Out : Outport  Port=8  VectorParamsAs1DForOutWhenUnconnected=off
  AutoRestartFFT_Out : Outport  Port=9  VectorParamsAs1DForOutWhenUnconnected=off
  ResetSymbol_Out : Outport  Port=10  VectorParamsAs1DForOutWhenUnconnected=off
  ResetFFT_Out : Outport  Port=11  VectorParamsAs1DForOutWhenUnconnected=off
  OutputGain_Out : Outport  Port=12  VectorParamsAs1DForOutWhenUnconnected=off
  ResetTime_Out : Outport  Port=13  VectorParamsAs1DForOutWhenUnconnected=off
  PacketSizeTime_Out : Outport  Port=14  VectorParamsAs1DForOutWhenUnconnected=off
  AutoRestartTime_Out : Outport  Port=15  VectorParamsAs1DForOutWhenUnconnected=off
  TransferTime_Out : Outport  Port=16  VectorParamsAs1DForOutWhenUnconnected=off
  SimulateInterface_Out : Outport  Port=17  VectorParamsAs1DForOutWhenUnconnected=off
  BypassGain_Out : Outport  Port=18  VectorParamsAs1DForOutWhenUnconnected=off
  RF_ch_sel_Out : Outport  Port=19  VectorParamsAs1DForOutWhenUnconnected=off
  wires:
  Enable/1 -> Slice/1
  LFSR_rst_In/1 -> LFSR_rst/1
  LFSR_rst/1 -> Slice1/1
  PacketSizeRF_In/1 -> PacketSizeRF/1
  Enable_In/1 -> Enable/1
  Slice/1 -> Enable_Out/1
  Slice1/1 -> LFSR_rst_Out/1
  PacketSizeRF/1 -> PacketSizeRF_Out/1
  PacketSizeFFT/1 -> PacketSizeFFT_Out/1
  PacketSizeFFT_In/1 -> PacketSizeFFT/1
  PacketSizeSymbol_In/1 -> PacketSizeSymbol/1
  PacketSizeSymbol/1 -> PacketSizeSymbol_Out/1
  TransferFFT/1 -> Slice2/1
  TransferFFT_In/1 -> TransferFFT/1
  TransferSymbol_In/1 -> TransferSymbol/1
  TransferSymbol/1 -> Slice3/1
  AutoRestartSymbol/1 -> Slice4/1
  AutoRestartSymbol_In/1 -> AutoRestartSymbol/1
  AutoRestartFFT_In/1 -> AutoRestartFFT/1
  AutoRestartFFT/1 -> Slice5/1
  Slice2/1 -> TransferFFT_Out/1
  Slice3/1 -> TransferSymbol_Out/1
  Slice4/1 -> AutoRestartSymbol_Out/1
  Slice5/1 -> AutoRestartFFT_Out/1
  ResetFFT/1 -> Slice7/1
  ResetFFT_In/1 -> ResetFFT/1
  ResetSymbol_In/1 -> ResetSymbol/1
  ResetSymbol/1 -> Slice6/1
  Slice6/1 -> ResetSymbol_Out/1
  Slice7/1 -> ResetFFT_Out/1
  OutputGain/1 -> Reinterpret/1
  OutputGain_In/1 -> OutputGain/1
  Slice8/1 -> ResetTime_Out/1
  ResetTime_In/1 -> ResetTime/1
  ResetTime/1 -> Slice8/1
  Slice9/1 -> AutoRestartTime_Out/1
  AutoRestartTime_In/1 -> AutoRestartTime/1
  AutoRestartTime/1 -> Slice9/1
  Slice10/1 -> TransferTime_Out/1
  TransferTime/1 -> Slice10/1
  TransferTime_In/1 -> TransferTime/1
  PacketSizeTime/1 -> PacketSizeTime_Out/1
  PacketSizeTime_In/1 -> PacketSizeTime/1
  Reinterpret/1 -> OutputGain_Out/1
  SimulateInterface_In/1 -> SimulateInterface/1
  SimulateInterface/1 -> Slice11/1
  Slice11/1 -> SimulateInterface_Out/1
  Slice12/1 -> BypassGain_Out/1
  BypassGain/1 -> Slice12/1
  BypassGain_In/1 -> BypassGain/1
  Slice13/1 -> RF_ch_sel_Out/1
  RF_ch_sel_In/1 -> RF_ch_sel/1
  RF_ch_sel/1 -> Slice13/1

== system AXI_QPSK_Tx/AXI_QPSK_Generator/M_AXIS_CH0 ==
  tdata_in : Inport
  tvalid_in : Inport  Port=2
  tlast_in : Inport  Port=3
  tready_in : Inport  Port=4
  m_rf0_axis_tdata : hdlBasic/Gateway Out  inherit_from_input=on  hdl_port=on  rows=1  columns=1  UseAsDAC=off  DACChannel='1'  interface=None  automatic_assignment=on  address_offset=hex2dec('00')  intf_name=''  intf_description=''  timing_constraint=None  locs_specified=off  LOCs={}  io_standard={}  XmcBlockStatus=1  maskContainerNames=group4  block_type=gatewayout  block_config=sysgen:gateway_out_config  block_width_w=590  block_height_w=620  block_width=620  block_height=750
  m_rf0_axis_tlast : hdlBasic/Gateway Out  inherit_from_input=off  hdl_port=on  rows=1  columns=1  UseAsDAC=off  DACChannel='1'  interface=None  automatic_assignment=on  address_offset=hex2dec('00')  intf_name=''  intf_description=''  timing_constraint=None  locs_specified=off  LOCs={}  io_standard={}  XmcBlockStatus=1  maskContainerNames=group4  block_type=gatewayout  block_config=sysgen:gateway_out_config  block_width_w=590  block_height_w=620  block_width=620  block_height=750
  m_rf0_axis_tready : hdlBasic/Gateway In  gui_display_data_type=Boolean  arith_type=Boolean  n_bits=16  bin_pt=14  preci_type=Single  exp_width=8  frac_width=24  rows=1  columns=1  quantization="Round  (unbiased: +/- Inf)"  overflow=Saturate  period=1/(fCIC)  UseAsADC=off  ADCChannel='1'  interface=None  automatic_assignment=on  address_offset=hex2dec('00')  intf_name=''  intf_description=''  default_value=0  timing_constraint=None  locs_specified=off  LOCs={}  io_standard={}  inherit_from_input=off  hdl_port=on  XmcBlockStatus=1  maskContainerNames=group4  block_type=gatewayin  block_config=sysgen:gateway_in_config  block_width_w=590  block_height_w=620  block_width=640  block_height=850
  m_rf0_axis_tvalid : hdlBasic/Gateway Out  inherit_from_input=off  hdl_port=on  rows=1  columns=1  UseAsDAC=off  DACChannel='1'  interface=None  automatic_assignment=on  address_offset=hex2dec('00')  intf_name=''  intf_description=''  timing_constraint=None  locs_specified=off  LOCs={}  io_standard={}  XmcBlockStatus=1  maskContainerNames=group4  block_type=gatewayout  block_config=sysgen:gateway_out_config  block_width_w=590  block_height_w=620  block_width=620  block_height=750
  tdata_out : Outport  VectorParamsAs1DForOutWhenUnconnected=off
  tvalid_out : Outport  Port=2  VectorParamsAs1DForOutWhenUnconnected=off
  tlast_out : Outport  Port=3  VectorParamsAs1DForOutWhenUnconnected=off
  tready_out : Outport  Port=4  VectorParamsAs1DForOutWhenUnconnected=off
  wires:
  tlast_in/1 -> m_rf0_axis_tlast/1
  m_rf0_axis_tlast/1 -> tlast_out/1
  m_rf0_axis_tready/1 -> tready_out/1
  tvalid_in/1 -> m_rf0_axis_tvalid/1
  m_rf0_axis_tvalid/1 -> tvalid_out/1
  tdata_in/1 -> m_rf0_axis_tdata/1
  m_rf0_axis_tdata/1 -> tdata_out/1
  tready_in/1 -> m_rf0_axis_tready/1

== system AXI_QPSK_Tx/AXI_QPSK_Generator/M_AXIS_CH1 ==
  tdata_in : Inport
  tvalid_in : Inport  Port=2
  tlast_in : Inport  Port=3
  tready_in : Inport  Port=4
  m_rf1_axis_tdata : hdlBasic/Gateway Out  inherit_from_input=on  hdl_port=on  rows=1  columns=1  UseAsDAC=off  DACChannel='1'  interface=None  automatic_assignment=on  address_offset=hex2dec('00')  intf_name=''  intf_description=''  timing_constraint=None  locs_specified=off  LOCs={}  io_standard={}  XmcBlockStatus=1  maskContainerNames=group4  block_type=gatewayout  block_config=sysgen:gateway_out_config  block_width_w=590  block_height_w=620  block_width=620  block_height=750
  m_rf1_axis_tlast : hdlBasic/Gateway Out  inherit_from_input=off  hdl_port=on  rows=1  columns=1  UseAsDAC=off  DACChannel='1'  interface=None  automatic_assignment=on  address_offset=hex2dec('00')  intf_name=''  intf_description=''  timing_constraint=None  locs_specified=off  LOCs={}  io_standard={}  XmcBlockStatus=1  maskContainerNames=group4  block_type=gatewayout  block_config=sysgen:gateway_out_config  block_width_w=590  block_height_w=620  block_width=620  block_height=750
  m_rf1_axis_tready : hdlBasic/Gateway In  gui_display_data_type=Boolean  arith_type=Boolean  n_bits=16  bin_pt=14  preci_type=Single  exp_width=8  frac_width=24  rows=1  columns=1  quantization="Round  (unbiased: +/- Inf)"  overflow=Saturate  period=1/(fCIC)  UseAsADC=off  ADCChannel='1'  interface=None  automatic_assignment=on  address_offset=hex2dec('00')  intf_name=''  intf_description=''  default_value=0  timing_constraint=None  locs_specified=off  LOCs={}  io_standard={}  inherit_from_input=off  hdl_port=on  XmcBlockStatus=1  maskContainerNames=group4  block_type=gatewayin  block_config=sysgen:gateway_in_config  block_width_w=590  block_height_w=620  block_width=640  block_height=850
  m_rf1_axis_tvalid : hdlBasic/Gateway Out  inherit_from_input=off  hdl_port=on  rows=1  columns=1  UseAsDAC=off  DACChannel='1'  interface=None  automatic_assignment=on  address_offset=hex2dec('00')  intf_name=''  intf_description=''  timing_constraint=None  locs_specified=off  LOCs={}  io_standard={}  XmcBlockStatus=1  maskContainerNames=group4  block_type=gatewayout  block_config=sysgen:gateway_out_config  block_width_w=590  block_height_w=620  block_width=620  block_height=750
  tdata_out : Outport  VectorParamsAs1DForOutWhenUnconnected=off
  tvalid_out : Outport  Port=2  VectorParamsAs1DForOutWhenUnconnected=off
  tlast_out : Outport  Port=3  VectorParamsAs1DForOutWhenUnconnected=off
  tready_out : Outport  Port=4  VectorParamsAs1DForOutWhenUnconnected=off
  wires:
  tlast_in/1 -> m_rf1_axis_tlast/1
  m_rf1_axis_tlast/1 -> tlast_out/1
  m_rf1_axis_tready/1 -> tready_out/1
  tvalid_in/1 -> m_rf1_axis_tvalid/1
  m_rf1_axis_tvalid/1 -> tvalid_out/1
  tdata_in/1 -> m_rf1_axis_tdata/1
  m_rf1_axis_tdata/1 -> tdata_out/1
  tready_in/1 -> m_rf1_axis_tready/1

== system AXI_QPSK_Tx/AXI_QPSK_Generator/M_AXIS_CH2 ==
  tdata_in : Inport
  tvalid_in : Inport  Port=2
  tlast_in : Inport  Port=3
  tready_in : Inport  Port=4
  m_rf2_axis_tdata : hdlBasic/Gateway Out  inherit_from_input=on  hdl_port=on  rows=1  columns=1  UseAsDAC=off  DACChannel='1'  interface=None  automatic_assignment=on  address_offset=hex2dec('00')  intf_name=''  intf_description=''  timing_constraint=None  locs_specified=off  LOCs={}  io_standard={}  XmcBlockStatus=1  maskContainerNames=group4  block_type=gatewayout  block_config=sysgen:gateway_out_config  block_width_w=590  block_height_w=620  block_width=620  block_height=750
  m_rf2_axis_tlast : hdlBasic/Gateway Out  inherit_from_input=off  hdl_port=on  rows=1  columns=1  UseAsDAC=off  DACChannel='1'  interface=None  automatic_assignment=on  address_offset=hex2dec('00')  intf_name=''  intf_description=''  timing_constraint=None  locs_specified=off  LOCs={}  io_standard={}  XmcBlockStatus=1  maskContainerNames=group4  block_type=gatewayout  block_config=sysgen:gateway_out_config  block_width_w=590  block_height_w=620  block_width=620  block_height=750
  m_rf2_axis_tready : hdlBasic/Gateway In  gui_display_data_type=Boolean  arith_type=Boolean  n_bits=16  bin_pt=14  preci_type=Single  exp_width=8  frac_width=24  rows=1  columns=1  quantization="Round  (unbiased: +/- Inf)"  overflow=Saturate  period=1/(fCIC)  UseAsADC=off  ADCChannel='1'  interface=None  automatic_assignment=on  address_offset=hex2dec('00')  intf_name=''  intf_description=''  default_value=0  timing_constraint=None  locs_specified=off  LOCs={}  io_standard={}  inherit_from_input=off  hdl_port=on  XmcBlockStatus=1  maskContainerNames=group4  block_type=gatewayin  block_config=sysgen:gateway_in_config  block_width_w=590  block_height_w=620  block_width=640  block_height=850
  m_rf2_axis_tvalid : hdlBasic/Gateway Out  inherit_from_input=off  hdl_port=on  rows=1  columns=1  UseAsDAC=off  DACChannel='1'  interface=None  automatic_assignment=on  address_offset=hex2dec('00')  intf_name=''  intf_description=''  timing_constraint=None  locs_specified=off  LOCs={}  io_standard={}  XmcBlockStatus=1  maskContainerNames=group4  block_type=gatewayout  block_config=sysgen:gateway_out_config  block_width_w=590  block_height_w=620  block_width=620  block_height=750
  tdata_out : Outport  VectorParamsAs1DForOutWhenUnconnected=off
  tvalid_out : Outport  Port=2  VectorParamsAs1DForOutWhenUnconnected=off
  tlast_out : Outport  Port=3  VectorParamsAs1DForOutWhenUnconnected=off
  tready_out : Outport  Port=4  VectorParamsAs1DForOutWhenUnconnected=off
  wires:
  tlast_in/1 -> m_rf2_axis_tlast/1
  m_rf2_axis_tlast/1 -> tlast_out/1
  m_rf2_axis_tready/1 -> tready_out/1
  tvalid_in/1 -> m_rf2_axis_tvalid/1
  m_rf2_axis_tvalid/1 -> tvalid_out/1
  tdata_in/1 -> m_rf2_axis_tdata/1
  m_rf2_axis_tdata/1 -> tdata_out/1
  tready_in/1 -> m_rf2_axis_tready/1

== system AXI_QPSK_Tx/AXI_QPSK_Generator/M_AXIS_CH3 ==
  tdata_in : Inport
  tvalid_in : Inport  Port=2
  tlast_in : Inport  Port=3
  tready_in : Inport  Port=4
  m_rf3_axis_tdata : hdlBasic/Gateway Out  inherit_from_input=on  hdl_port=on  rows=1  columns=1  UseAsDAC=off  DACChannel='1'  interface=None  automatic_assignment=on  address_offset=hex2dec('00')  intf_name=''  intf_description=''  timing_constraint=None  locs_specified=off  LOCs={}  io_standard={}  XmcBlockStatus=1  maskContainerNames=group4  block_type=gatewayout  block_config=sysgen:gateway_out_config  block_width_w=590  block_height_w=620  block_width=620  block_height=750
  m_rf3_axis_tlast : hdlBasic/Gateway Out  inherit_from_input=off  hdl_port=on  rows=1  columns=1  UseAsDAC=off  DACChannel='1'  interface=None  automatic_assignment=on  address_offset=hex2dec('00')  intf_name=''  intf_description=''  timing_constraint=None  locs_specified=off  LOCs={}  io_standard={}  XmcBlockStatus=1  maskContainerNames=group4  block_type=gatewayout  block_config=sysgen:gateway_out_config  block_width_w=590  block_height_w=620  block_width=620  block_height=750
  m_rf3_axis_tready : hdlBasic/Gateway In  gui_display_data_type=Boolean  arith_type=Boolean  n_bits=16  bin_pt=14  preci_type=Single  exp_width=8  frac_width=24  rows=1  columns=1  quantization="Round  (unbiased: +/- Inf)"  overflow=Saturate  period=1/(fCIC)  UseAsADC=off  ADCChannel='1'  interface=None  automatic_assignment=on  address_offset=hex2dec('00')  intf_name=''  intf_description=''  default_value=0  timing_constraint=None  locs_specified=off  LOCs={}  io_standard={}  inherit_from_input=off  hdl_port=on  XmcBlockStatus=1  maskContainerNames=group4  block_type=gatewayin  block_config=sysgen:gateway_in_config  block_width_w=590  block_height_w=620  block_width=640  block_height=850
  m_rf3_axis_tvalid : hdlBasic/Gateway Out  inherit_from_input=off  hdl_port=on  rows=1  columns=1  UseAsDAC=off  DACChannel='1'  interface=None  automatic_assignment=on  address_offset=hex2dec('00')  intf_name=''  intf_description=''  timing_constraint=None  locs_specified=off  LOCs={}  io_standard={}  XmcBlockStatus=1  maskContainerNames=group4  block_type=gatewayout  block_config=sysgen:gateway_out_config  block_width_w=590  block_height_w=620  block_width=620  block_height=750
  tdata_out : Outport  VectorParamsAs1DForOutWhenUnconnected=off
  tvalid_out : Outport  Port=2  VectorParamsAs1DForOutWhenUnconnected=off
  tlast_out : Outport  Port=3  VectorParamsAs1DForOutWhenUnconnected=off
  tready_out : Outport  Port=4  VectorParamsAs1DForOutWhenUnconnected=off
  wires:
  tlast_in/1 -> m_rf3_axis_tlast/1
  m_rf3_axis_tlast/1 -> tlast_out/1
  m_rf3_axis_tready/1 -> tready_out/1
  tvalid_in/1 -> m_rf3_axis_tvalid/1
  m_rf3_axis_tvalid/1 -> tvalid_out/1
  tdata_in/1 -> m_rf3_axis_tdata/1
  m_rf3_axis_tdata/1 -> tdata_out/1
  tready_in/1 -> m_rf3_axis_tready/1

== system AXI_QPSK_Tx/AXI_QPSK_Generator/M_AXIS_FFT ==
  tdata_in : Inport
  tvalid_in : Inport  Port=2
  tlast_in : Inport  Port=3
  tready_in : Inport  Port=4
  m_fft_axis_tdata : hdlBasic/Gateway Out  inherit_from_input=on  hdl_port=on  rows=1  columns=1  UseAsDAC=off  DACChannel='1'  interface=None  automatic_assignment=on  address_offset=hex2dec('00')  intf_name=''  intf_description=''  timing_constraint=None  locs_specified=off  LOCs={}  io_standard={}  XmcBlockStatus=1  maskContainerNames=group4  block_type=gatewayout  block_config=sysgen:gateway_out_config  block_width_w=590  block_height_w=620  block_width=620  block_height=750
  m_fft_axis_tlast : hdlBasic/Gateway Out  inherit_from_input=off  hdl_port=on  rows=1  columns=1  UseAsDAC=off  DACChannel='1'  interface=None  automatic_assignment=on  address_offset=hex2dec('00')  intf_name=''  intf_description=''  timing_constraint=None  locs_specified=off  LOCs={}  io_standard={}  XmcBlockStatus=1  maskContainerNames=group4  block_type=gatewayout  block_config=sysgen:gateway_out_config  block_width_w=590  block_height_w=620  block_width=620  block_height=750
  m_fft_axis_tready : hdlBasic/Gateway In  gui_display_data_type=Boolean  arith_type=Boolean  n_bits=16  bin_pt=14  preci_type=Single  exp_width=8  frac_width=24  rows=1  columns=1  quantization="Round  (unbiased: +/- Inf)"  overflow=Saturate  period=1/(fCIC)  UseAsADC=off  ADCChannel='1'  interface=None  automatic_assignment=on  address_offset=hex2dec('00')  intf_name=''  intf_description=''  default_value=0  timing_constraint=None  locs_specified=off  LOCs={}  io_standard={}  inherit_from_input=off  hdl_port=on  XmcBlockStatus=1  maskContainerNames=group4  block_type=gatewayin  block_config=sysgen:gateway_in_config  block_width_w=590  block_height_w=620  block_width=640  block_height=850
  m_fft_axis_tvalid : hdlBasic/Gateway Out  inherit_from_input=off  hdl_port=on  rows=1  columns=1  UseAsDAC=off  DACChannel='1'  interface=None  automatic_assignment=on  address_offset=hex2dec('00')  intf_name=''  intf_description=''  timing_constraint=None  locs_specified=off  LOCs={}  io_standard={}  XmcBlockStatus=1  maskContainerNames=group4  block_type=gatewayout  block_config=sysgen:gateway_out_config  block_width_w=590  block_height_w=620  block_width=620  block_height=750
  tdata_out : Outport  VectorParamsAs1DForOutWhenUnconnected=off
  tvalid_out : Outport  Port=2  VectorParamsAs1DForOutWhenUnconnected=off
  tlast_out : Outport  Port=3  VectorParamsAs1DForOutWhenUnconnected=off
  tready_out : Outport  Port=4  VectorParamsAs1DForOutWhenUnconnected=off
  wires:
  tready_in/1 -> m_fft_axis_tready/1
  m_fft_axis_tdata/1 -> tdata_out/1
  tdata_in/1 -> m_fft_axis_tdata/1
  m_fft_axis_tvalid/1 -> tvalid_out/1
  tvalid_in/1 -> m_fft_axis_tvalid/1
  m_fft_axis_tready/1 -> tready_out/1
  m_fft_axis_tlast/1 -> tlast_out/1
  tlast_in/1 -> m_fft_axis_tlast/1
